simulink model "grasp_object"  (R2023a)
settings: Solver=FixedStepDiscrete  StartTime=0.0  StopTime=inf  FixedStep=0.001  RelTol=1e-3  EnableMultiTasking=on
PreLoadFcn:
  | frs = FrankaRobotSettings;
libraries: franka_simulink_library x4, simulink x1
settings Model: SimulationMode=external  ExtModeTrigDuration=10000  Creator=vasi_ko  LastModifiedBy=kvasios
settings SolverCC: AlgebraicLoopSolver=TrustRegion
settings DataIOCC: LimitDataPoints=on  SaveFormat=Array  ReturnWorkspaceOutputs=off
settings OptimizationCC: DefaultParameterBehavior=Inlined  EnhancedBackFolding=on  PassReuseOutputArgsThreshold=0  OptimizeBlockOrder=speed  DifferentSizesBufferReuse=on  OptimizationCustomize=off
settings DebuggingCC: SolverPrmCheckMsg=warning  ParameterTunabilityLossMsg=error  UnconnectedInputMsg=warning  UnconnectedOutputMsg=warning  UnconnectedLineMsg=warning  SFUnexpectedBacktrackingDiag=warning  SFNoUnconditionalDefaultTransitionDiag=warning  SFExecutionAtInitializationDiag=none  ArithmeticOperatorsInVariantConditions=warning
settings ModelReferenceCC: EnableRefExpFcnMdlSchedulingChecks=on  PropagateSignalLabelsOutOfModel=off
settings SFSimCC: SimUseLocalCustomCode=off  MATLABDynamicMemAlloc=off  CustomCodeUndefinedFunction=UseInterfaceOnly  SimTargetLang=C++
settings RTWCC: RTWVerbose=off  RTWUseLocalCustomCode=off  BuildConfiguration=Faster Runs  TargetLang=C++  DLArmComputeVersion=19.05
settings CodeAppCC: ForceParamTrailComments=on  OperatorAnnotations=on
settings ConfigComp: CovMetricSettings=dw  CovSaveCumulativeToWorkspaceVar=on  CovSaveSingleToWorkspaceVar=on  CovExternalEMLEnable=off  CovSFcnEnable=off

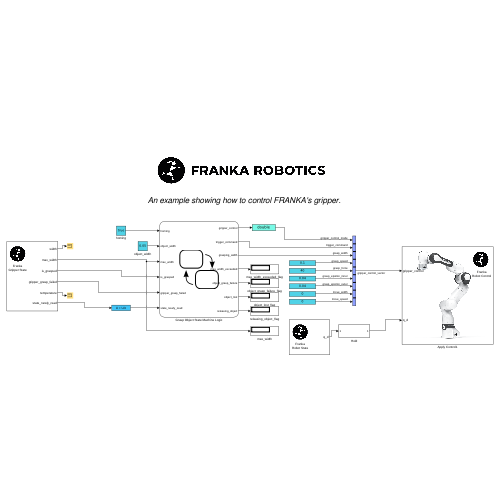
[thumbnail: Simulink's stored preview of the top-level diagram]
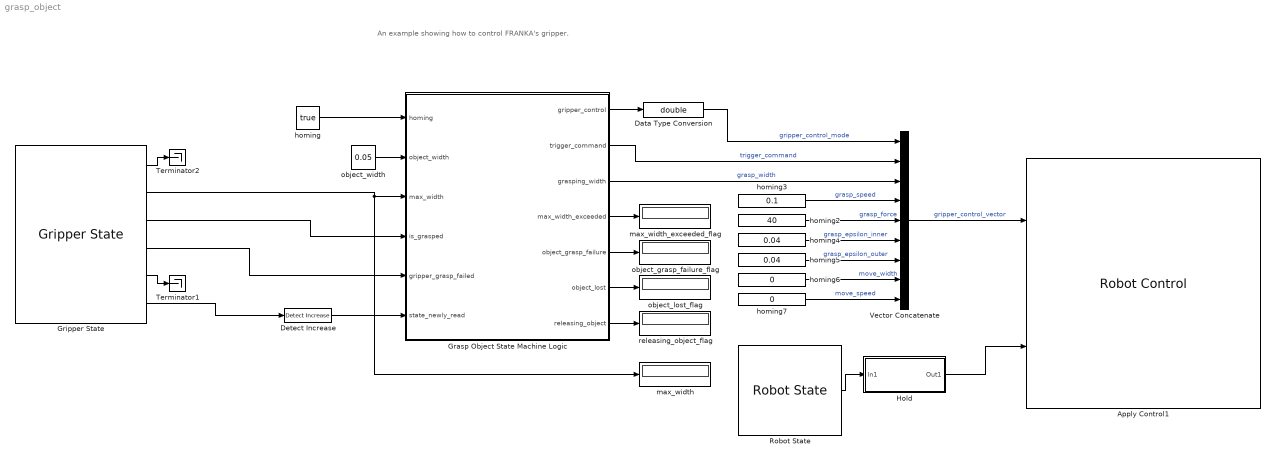
== system grasp_object ==
  note: An example showing how to control FRANKA's gripper.
  Apply Control1 : franka_simulink_library/Robot Control  robot_ip=frs.robot_ip  gripper_selection=Franka Gripper  control_mode=Joint Positions - Internal Controller Mode  controller_choice=Joint Impedance Controller  joint_impedance=frs.joint_impedance_stiffness  cartesian_impedance=[3000, 3000, 3000, 300, 300, 300]  rate_limiter=on  cuttoff_frequency=frs.cutoff_frequency  elbow_control=off  collision_thresholds=frs.collision_thresholds.getAs1DArray  load_inertia=frs.load_inertia.getAs1DArray  NE_T_EE=frs.NE_T_EE(:)  EE_T_K=frs.EE_T_K(:)  init_joint_configuration_req=on  init_joint_configuration=frs.home_configuration
      settings: SourceProductName=Franka Robotics Simulink Support Package
  Data Type Conversion : DataTypeConversion  OutDataTypeStr=double  SaturateOnIntegerOverflow=off  RndMeth=Floor
  Detect Increase : simulink/Logic and Bit Operations/Detect Increase  vinit=0.0  OutDataTypeStr=boolean
  Grasp Object State Machine Logic : Stateflow chart  TreatAsAtomicUnit=on
  Gripper State : franka_simulink_library/Gripper State  robot_ip=frs.robot_ip
      settings: SourceProductName=Franka Robotics Simulink Support Package
  Hold : Subsystem
  Robot State : franka_simulink_library/Robot State  robot_ip=frs.robot_ip  signals_requested='q_d'
      settings: SourceProductName=Franka Robotics Simulink Support Package
  Terminator1 : Terminator
  Terminator2 : Terminator
  Vector Concatenate : Concatenate  NumInputs=9
  homing : Constant  Value=true
  homing2 : Constant  Value=40
  homing3 : Constant  Value=0.1
  homing4 : Constant  Value=0.04
  homing5 : Constant  Value=0.04
  homing6 : Constant  Value=0
  homing7 : Constant  Value=0
  max_width : Display
  max_width_exceeded_flag : Display
  object_grasp_failure_flag : Display
  object_lost_flag : Display
  object_width : Constant  Value=0.05
  releasing_object_flag : Display
  wires:
  homing/1 -> Grasp Object State Machine Logic/1(homing)
  Gripper State/2 -> max_width/1, Grasp Object State Machine Logic/3(max_width)
  Gripper State/3 -> Grasp Object State Machine Logic/4(is_grasped)
  Detect Increase/1 -> Grasp Object State Machine Logic/6(state_newly_read)
  Gripper State/6 -> Detect Increase/1
  Grasp Object State Machine Logic/1(gripper_control) -> Data Type Conversion/1
  Grasp Object State Machine Logic/4(max_width_exceeded) -> max_width_exceeded_flag/1
  Grasp Object State Machine Logic/5(object_grasp_failure) -> object_grasp_failure_flag/1
  Grasp Object State Machine Logic/6(object_lost) -> object_lost_flag/1
  Grasp Object State Machine Logic/7(releasing_object) -> releasing_object_flag/1
  Gripper State/4 -> Grasp Object State Machine Logic/5(gripper_grasp_failed)
  Gripper State/1 -> Terminator2/1
  Gripper State/5 -> Terminator1/1
  Vector Concatenate/1 -> Apply Control1/1  "gripper_control_vector"
  Data Type Conversion/1 -> Vector Concatenate/1  "gripper_control_mode"
  Grasp Object State Machine Logic/3(grasping_width) -> Vector Concatenate/3  "grasp_width"
  homing3/1 -> Vector Concatenate/4  "grasp_speed"
  homing2/1 -> Vector Concatenate/5  "grasp_force"
  homing4/1 -> Vector Concatenate/6  "grasp_epsilon_inner"
  homing5/1 -> Vector Concatenate/7  "grasp_epsilon_outer"
  homing6/1 -> Vector Concatenate/8  "move_width"
  homing7/1 -> Vector Concatenate/9  "move_speed"
  object_width/1 -> Grasp Object State Machine Logic/2(object_width)
  Grasp Object State Machine Logic/2(trigger_command) -> Vector Concatenate/2  "trigger_command"
  Robot State/1 -> Hold/1(In1)
  Hold/1(Out1) -> Apply Control1/2

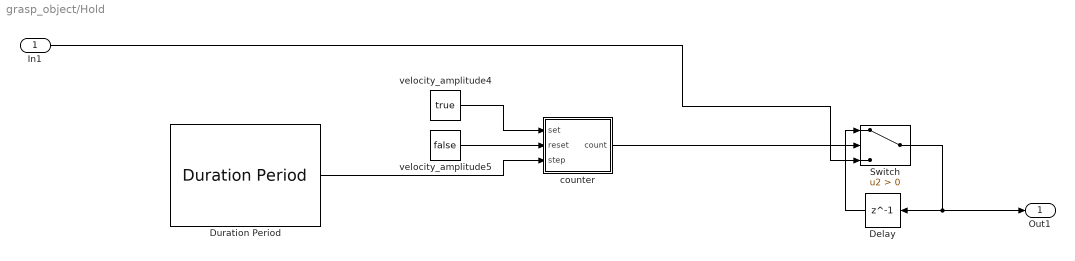
== system grasp_object/Hold ==
  In1 : Inport
  Delay : Delay  DelayLength=1
  Duration Period : franka_simulink_library/Duration Period  robot_ip=frs.robot_ip
      settings: SourceProductName=Franka Robotics Simulink Support Package
  Switch : Switch  Criteria=u2 > Threshold  SaturateOnIntegerOverflow=off  InputSameDT=off
  counter : Subsystem
  velocity_amplitude4 : Constant  Value=true  VectorParams1D=off
  velocity_amplitude5 : Constant  Value=false  VectorParams1D=off
  Out1 : Outport
  wires:
  counter/1(count) -> Switch/2
  velocity_amplitude4/1 -> counter/1(set)
  velocity_amplitude5/1 -> counter/2(reset)
  In1/1 -> Switch/3
  Delay/1 -> Switch/1
  Switch/1 -> Out1/1, Delay/1
  Duration Period/1 -> counter/3(step)

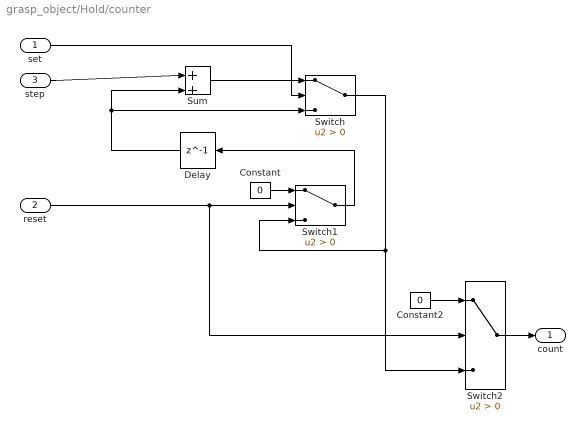
== system grasp_object/Hold/counter ==
  set : Inport  OutDataTypeStr=boolean
  reset : Inport  Port=2  OutDataTypeStr=boolean
  step : Inport  Port=3  OutDataTypeStr=double
  Constant : Constant  Value=0  OutDataTypeStr=double
  Constant2 : Constant  Value=0  OutDataTypeStr=double
  Delay : Delay  DelayLength=1  InitialCondition=0
  Sum : Sum  Inputs=|++
  Switch : Switch  Criteria=u2 > Threshold  SaturateOnIntegerOverflow=off  InputSameDT=off
  Switch1 : Switch  Criteria=u2 > Threshold  OutDataTypeStr=double  SaturateOnIntegerOverflow=off  InputSameDT=off
  Switch2 : Switch  Criteria=u2 > Threshold  OutDataTypeStr=double  SaturateOnIntegerOverflow=off  InputSameDT=off
  count : Outport  OutDataTypeStr=double  VectorParamsAs1DForOutWhenUnconnected=off
  wires:
  Switch2/1 -> count/1
  Constant2/1 -> Switch2/1
  Sum/1 -> Switch/1
  set/1 -> Switch/2
  Switch/1 -> Switch1/3, Switch2/3
  step/1 -> Sum/1
  Delay/1 -> Sum/2, Switch/3
  reset/1 -> Switch1/2, Switch2/2
  Constant/1 -> Switch1/1
  Switch1/1 -> Delay/1

== stateflow chart grasp_object/Grasp Object State Machine Logic ==
  state starting_point
  state gripper_control_activated
  state homing
    en:gripper_control = FrankaGripperControlModes.homing;
    trigger_command = trigger_command + 1;
  state read_state
    en:gripper_control = FrankaGripperControlModes.read_state;
    trigger_command = trigger_command + 1;
  state max_grasp_width_check
  state max_grasp_width_within_range
    en:max_width_exceeded = 0;
  state max_grasp_width_exceeded
    en:max_width_exceeded = 1;
  state grasp_object
    en:grasping_width = object_width;
    gripper_control = FrankaGripperControlModes.grasp;
    trigger_command = trigger_command + 1;
  state wait_grasp_command_update
  state grasp_succeeded
    en:object_grasp_failure = 0;
  state grasp_failed
    en:object_grasp_failure = 1;
  state read_state_2
    en:gripper_control = FrankaGripperControlModes.read_state;
    trigger_command = trigger_command + 1;
  state check_if_object_is_lost
  state object_lost
    en:object_lost = 1;
  state object_not_lost
    en:object_lost = 0;
  state releasing_object
    en:gripper_control = FrankaGripperControlModes.stop;
    trigger_command = trigger_command + 1;
  state fin
  (default) -> starting_point : {gripper_control = FrankaGripperControlModes.idle;
      | trigger_command = 0;
      | max_width_exceeded = 0;
      | object_grasp_failure = 0;
      | object_lost=0;
      | releasing_object=0}
  starting_point -> gripper_control_activated
  gripper_control_activated -> homing [order 1] : [homing]
  gripper_control_activated -> read_state [order 2] : [~homing]
  homing -> read_state : [state_newly_read]
  read_state -> max_grasp_width_check : [state_newly_read]
  max_grasp_width_check -> max_grasp_width_within_range [order 2] : [object_width<=max_width]
  max_grasp_width_check -> max_grasp_width_exceeded [order 1] : [object_width>max_width]
  max_grasp_width_within_range -> grasp_object : after(5,sec)
  grasp_object -> wait_grasp_command_update : [state_newly_read]
  wait_grasp_command_update -> grasp_failed [order 2] : [gripper_grasp_failed]
  wait_grasp_command_update -> grasp_succeeded [order 1] : [~gripper_grasp_failed]
  grasp_succeeded -> read_state_2 : after(3,sec)
  read_state_2 -> check_if_object_is_lost : [state_newly_read]
  check_if_object_is_lost -> object_lost [order 1] : [~is_grasped]
  check_if_object_is_lost -> object_not_lost [order 2] : [is_grasped]
  object_not_lost -> releasing_object : {releasing_object = 1;}
  releasing_object -> fin : [state_newly_read]
  data: gripper_control output; trigger_command output; grasping_width output; homing input; object_width input; max_width input; is_grasped input; gripper_grasp_failed input; state_newly_read input; max_width_exceeded output; object_grasp_failure output; object_lost output; releasing_object output
